simulink model "GPCA_Extension"  (Simulink 7.9)
settings: Solver=ode45  StartTime=0.0  StopTime=inf  RelTol=1e-3
PreLoadFcn:
  | GPCA_Bus_Def
InitFcn:
  | script
values from neighbouring files (symbols this model uses):
  GOutputEvents = [0 0 0 0 0 0 0 0 0 0 0 0 0 0 0 0 0 0 0 0 0]    [script.m]
  GProgrammedDoseRate = 0    [script.m]
  GProgrammedVTBI = 0    [script.m]
libraries: simulink x6
(part 2 of 3)

== stateflow chart GPCA Software Controller/StateChanger ==
  state x = displayBolusInfo [function]
    (junction 152) -> (junction 154) [order 1] : [infuStatus.isBolusInProgress == 1]{bolusing := 1; ml.GAlrmMsg = MSG_BOLUSGRANT; }
    (default) -> (junction 152)
    (junction 152) -> (junction 153) [order 2] : [infuStatus.isBolusInProgress == 0]{ml.GAlrmMsg = MSG_BOLUSDENIED; }
  state x1 = enterinto(stateId) [function]
    (junction 88) -> (junction 89) : {x1 := stateId;}
    (default) -> (junction 88) : {O_CurrentState := stateId;}
  state x = resumeInfusion [function]
    (junction 200) -> (junction 109) : {O_InfusionInProgress := 1;
        |  O_InfusionPaused := 0;
        |  O_BolusRequested := 0;}
    (default) -> (junction 199)
    (junction 199) -> (junction 200) : {infusing := 1; bolusing := 0;}
  state x = warning [function]
    (junction 127) -> (junction 108) [order 2] : [ErrCond == 17]{ml.GAlrmMsg = MSG_LOWRESR;}
    (junction 127) -> (junction 128) [order 1] : [ErrCond == 16]{ml.GAlrmMsg = MSG_FLOWRATEVARY;}
    (junction 127) -> (junction 115) [order 4] : [ErrCond == 19]{ml.GAlrmMsg = MSG_LOGERR; }
    (junction 127) -> (junction 120) [order 11] : [ErrCond == 26]{ml.GAlrmMsg = MSG_DANGERAP;}
    (junction 127) -> (junction 121) [order 3] : [ErrCond ==18]{ml.GAlrmMsg = MSG_PAUSELONG;}
    (junction 127) -> (junction 122) [order 5] : [ErrCond==20]{ml.GAlrmMsg = MSG_LOWBATT; }
    (junction 127) -> (junction 123) [order 6] : [ErrCond==21]{ml.GAlrmMsg = MSG_WRNBATTERYCHARGE;}
    (junction 127) -> (junction 125) [order 7] : [ErrCond==22]{ml.GAlrmMsg = MSG_VOLTOUTRANGE;}
    (junction 127) -> (junction 126) [order 8] : [ErrCond==23]{ml.GAlrmMsg = MSG_PUMPOVERHEAT;}
    (default) -> (junction 127) : {O_AlarmCond := ErrCond;}
    (junction 127) -> (junction 131) [order 9] : [ErrCond==24]{ml.GAlrmMsg = MSG_DANGERENVTEMP;}
    (junction 127) -> (junction 137) [order 10] : [ErrCond == 25]{ml.GAlrmMsg = MSG_DANGERHUMD;}
  state x = initInfusion [function]
    (default) -> (junction 138)
    (junction 138) -> (junction 139) : { bolusing := 0; infusing := 0; doseRate := 0; vtbi := 0;
        |   resetInfusionInstructions();}
  state x = checkDoseRate(iRate) [function]
    (junction 188) -> (junction 173) [order 2] : [iRate <= drugLibInfo.doseRateUpperHardLimit && iRate >= drugLibInfo.doseRateLowerHardLimit]
    (junction 173) -> (junction 148) [order 1] : [iRate > drugLibInfo.doseRateUpperSoftLimit || iRate < drugLibInfo.doseRateLowerSoftLimit]{ x := 1;}
    (junction 188) -> (junction 157) [order 1] : [iRate > drugLibInfo.doseRateUpperHardLimit || iRate < drugLibInfo.doseRateLowerHardLimit]{ x := 2;}
    (junction 173) -> (junction 91) [order 2] : [iRate <= drugLibInfo.doseRateUpperSoftLimit && iRate >= drugLibInfo.doseRateLowerSoftLimit]{ x:= 0;}
    (default) -> (junction 188)
  state x = clearAlrm (alrm) [function]
    (default) -> (junction 93) : {ClearCond := alrm;}
    (junction 93) -> (junction 94) : {E_AlarmClear;}
  state x = setPatientInfo [function]
    (default) -> (junction 167)
    (junction 167) -> (junction 169) : {O_PatientInfo.patientID := patientInfo.patientID;
        |  O_PatientInfo.patientAge := patientInfo.patientAge;
        |  O_PatientInfo.patientGender := patientInfo.patientGender;
        | O_PatientInfo.patientWeight := patientInfo.patientWeight;}
  state x = initPatientInfo [function]
    (junction 187) -> (junction 144) : { O_PatientInfo.patientID := 0;  O_PatientInfo.patientAge := 0;
        |   O_PatientInfo.patientGender := 0; O_PatientInfo.patientWeight := 0;}
    (default) -> (junction 187)
  state x = setDrugLibInfo [function]
    (junction 124) -> (junction 155) : { O_DrugLibInfo.drugConcentrationTypical = drugLibInfo.drugConcentrationTypical;
        |   O_DrugLibInfo.drugConcentrationUpperHardLimit = drugLibInfo.drugConcentrationUpperHardLimit;
        |   O_DrugLibInfo.drugConcentrationUpperSoftLimit = drugLibInfo.drugConcentrationUpperSoftLimit;
        |   O_DrugLibInfo.drugConcentrationLowerSoftLimit = drugLibInfo.drugConcentrationLowerSoftLimit;
        |   O_DrugLibInfo.drugConcentrationLowerHardLimit = drugLibInfo.drugConcentrationLowerHardLimit;}
    (default) -> (junction 132)
    (junction 132) -> (junction 143) : {O_DrugLibInfo.drugID = drugLibInfo.drugID; O_DrugLibInfo.amount = drugLibInfo.amount;}
    (junction 143) -> (junction 112) : { O_DrugLibInfo.doseRateTypical = drugLibInfo.doseRateTypical; O_DrugLibInfo.doseRateUnit = drugLibInfo.doseRateUnit;
        |   O_DrugLibInfo.doseRateUpperHardLimit = drugLibInfo.doseRateUpperHardLimit;
        |   O_DrugLibInfo.doseRateUpperSoftLimit = drugLibInfo.doseRateUpperSoftLimit;
        |   O_DrugLibInfo.doseRateLowerSoftLimit = drugLibInfo.doseRateLowerSoftLimit;
        |   O_DrugLibInfo.doseRateLowerHardLimit = drugLibInfo.doseRateLowerHardLimit;}
    (junction 112) -> (junction 124) : { O_DrugLibInfo.vtbiTypical = drugLibInfo.vtbiTypical; O_DrugLibInfo.vtbiUnit = drugLibInfo.vtbiUnit;
        |   O_DrugLibInfo.vtbiUpperHardLimit = drugLibInfo.vtbiUpperHardLimit;
        |   O_DrugLibInfo.vtbiUpperSoftLimit = drugLibInfo.vtbiUpperSoftLimit;
        |   O_DrugLibInfo.vtbiLowerSoftLimit = drugLibInfo.vtbiLowerSoftLimit;
        |   O_DrugLibInfo.vtbiLowerHardLimit = drugLibInfo.vtbiLowerHardLimit;}
  state x = setLOneMsg(fcond) [function]
    (default) -> (junction 98) : {O_AlarmCond := fcond;}
    (junction 98) -> (junction 99) [order 1] : [fcond==1]{ml.GAlrmMsg =MSG_OUTOFPOWER;}
    (junction 98) -> (junction 101) [order 3] : [fcond==3]{ml.GAlrmMsg = MSG_CPUFAILURE;}
    (junction 98) -> (junction 102) [order 4] : [fcond==4]{ml.GAlrmMsg = MSG_MEMORYCORRUPT;}
    (junction 98) -> (junction 103) [order 5] : [fcond==5]{ml.GAlrmMsg = MSG_PUMPTOOHOT;}
    (junction 98) -> (junction 104) [order 6] : [fcond==6]{ml.GAlrmMsg = MSG_WATCHDOGALERT;}
    (junction 98) -> (junction 100) [order 2] : [fcond==2]{ml.GAlrmMsg = MSG_REALTIMECLOCK;}
  state x = alrmLevel [function]
    (junction 96) -> (junction 184) [order 4] : [ErrCond == 0]{O_AlarmCond := ErrCond; x := 0;}
    (default) -> (junction 96)
    (junction 96) -> (junction 129) [order 1] : [ErrCond  > 0 && ErrCond <7] {O_AlarmCond := ErrCond; x:=1;}
    (junction 96) -> (junction 90) [order 2] : [ErrCond>=7 && ErrCond < 16]{O_AlarmCond := ErrCond; x:=2;}
    (junction 96) -> (junction 97) [order 3] : [ErrCond>=16]{O_AlarmCond := ErrCond; x:=3;}
  state x = setLTwoMsg(fCond) [function]
    (junction 111) -> (junction 107) [order 8] : [fCond==14]{ml.GAlrmMsg = MSG_PAUSETOOLONG;}
    (junction 111) -> (junction 105) [order 3] : [fCond==9]{ml.GAlrmMsg = MSG_OCCULUSION;}
    (junction 111) -> (junction 110) [order 9] : [fCond==15]{ml.GAlrmMsg = MSG_AIRINLINE;}
    (default) -> (junction 111) : {O_AlarmCond := fCond;}
    (junction 111) -> (junction 113) [order 1] : [fCond==7]{ml.GAlrmMsg = MSG_DOOROPEN;}
    (junction 111) -> (junction 114) [order 2] : [fCond==8]{ml.GAlrmMsg = MSG_EMPTYRESERVOIR;}
    (junction 111) -> (junction 116) [order 4] : [fCond==10]{ml.GAlrmMsg = MSG_OVERINFUSION;}
    (junction 111) -> (junction 117) [order 5] : [fCond==11]{ml.GAlrmMsg = MSG_UNDERINFUSION;}
    (junction 111) -> (junction 118) [order 6] : [fCond==12]{ml.GAlrmMsg = MSG_LESSTHANKVO;}
    (junction 111) -> (junction 119) [order 7] : [fCond==13]{ml.GAlrmMsg = MSG_RATEEXCEEDCAPACITY;}
  state x = bolusStatus [function]
    (default) -> (junction 134)
    (junction 134) -> (junction 135) [order 1] : [infuStatus.isBolusInProgress == 1]{bolusing := 1;
        | ml.GAlrmMsg = MSG_BOLUSGRANT;}
    (junction 134) -> (junction 136) [order 2] : [infuStatus.isBolusInProgress == 0]{bolusing := 0;
        | ml.GAlrmMsg = MSG_BOLUSDENIED;}
  state x = checkVTBI(inputVal) [function]
    (default) -> (junction 156)
    (junction 145) -> (junction 92) [order 2] : [(inputVal <= drugLibInfo.vtbiUpperSoftLimit) && (inputVal <= drugLibInfo.vtbiLowerSoftLimit)]{ x := 0;}
    (junction 145) -> (junction 95) [order 1] : [(inputVal > drugLibInfo.vtbiUpperSoftLimit) || (inputVal < drugLibInfo.vtbiLowerSoftLimit)]{ x := 1;}
    (junction 156) -> (junction 146) [order 1] : [(inputVal > drugLibInfo.vtbiUpperHardLimit) || (inputVal < drugLibInfo.vtbiLowerHardLimit)]{ x := 2;}
    (junction 156) -> (junction 145) [order 2] : [(inputVal <= drugLibInfo.vtbiUpperHardLimit) && (inputVal >= drugLibInfo.vtbiLowerHardLimit)]
  state x = calcFlowRate(iRate) [function]
    (junction 163) -> (junction 164) : {x := iRate /  drugInfo.drugConcentration;}
    (default) -> (junction 163)
  state x = checkDrugConcentration [function]
    (junction 174) -> (junction 172) [order 1] : [actualCon > upperHard || actualCon < lowerHard]{x := 2;}
    (junction 174) -> (junction 178) [order 2] : [actualCon <= upperHard && actualCon >= lowerHard]
    (default) -> (junction 174) : {actualCon := drugInfo.drugConcentration;
        | upperHard := drugLibInfo.drugConcentrationUpperHardLimit; upperSoft := drugLibInfo.drugConcentrationUpperSoftLimit;
        | lowerHard := drugLibInfo.drugConcentrationLowerHardLimit;  lowerSoft := drugLibInfo.drugConcentrationLowerSoftLimit;}
    (junction 178) -> (junction 176) [order 2] : [actualCon <= upperSoft && actualCon >= lowerSoft]{x := 0;}
    (junction 178) -> (junction 177) [order 1] : [actualCon > upperSoft || actualCon < lowerSoft]{x := 1;}
  state x = initDrugLib [function]
    (junction 168) -> (junction 166) : { O_DrugLibInfo.drugID := 0; O_DrugLibInfo.amount = 0; O_DrugLibInfo.diluentVolume := 0; O_DrugLibInfo.doseRateTypical := 0;
        |   O_DrugLibInfo.doseRateUpperHardLimit := 0; O_DrugLibInfo.doseRateUpperSoftLimit := 0; O_DrugLibInfo.doseRateLowerHardLimit := 0;
        |   O_DrugLibInfo.doseRateLowerSoftLimit := 0; O_DrugLibInfo.doseRateUnit := 0; O_DrugLibInfo.vtbiTypical := 0; O_DrugLibInfo.vtbiUpperHardLimit := 0;
        |   O_DrugLibInfo.vtbiUpperSoftLimit := 0; O_DrugLibInfo.vtbiLowerHardLimit := 0; O_DrugLibInfo.vtbiLowerSoftLimit := 0; O_DrugLibInfo.vtbiUnit :=0;
        |   O_DrugLibInfo.drugConcentrationTypical := 0; O_DrugLibInfo.drugConcentrationUpperHardLimit := 0; O_DrugLibInfo.drugConcentrationUpperSoftLimit := 0;
        |   O_DrugLibInfo.drugConcentrationLowerHardLimit := 0; O_DrugLibInfo.drugConcentrationLowerSoftLimit := 0;}
    (default) -> (junction 168)
  state x = init [function]
    (junction 159) -> (junction 130) : {temp := 0; tempx := 0; infusing :=0; bolusing :=0;}
    (default) -> (junction 183)
    (junction 183) -> (junction 159) : { ClearCond := 0; O_InfusionInProgress := 0; O_InfusionPaused := 0;
        |   O_BolusRequested := 0; O_ProgrammedVTBI := 0; O_ProgrammedFlowRate := 0; O_CurrentState := 0;
        |   O_AlarmCond := 0;  initDrugLib(); initPatientInfo();}
  state InfusionStateMachine
    state ConfirmPowerDown
      en: enterinto(2);
      ml.GMsgConStr := MSG_POWEROFF;
    state PowerOff
      en: enterinto(1);
      ex: ml.GMsgConStr = MSG_WELCOME;
    state POST
      en: enterinto(3);
      tempx := pumpConfigData.isPOSTSuccessful ;
    state ALM_POSTFailed
      en:  ml.GMsgConStr =MSG_POSTFAIL;
      enterinto(4);
    state InfusionInSession
      (history)
      state InfusionPaused
        en: enterinto(36);
        pauseInfusion();
        ml.GMsgConStr = MSG_INFUSIONPAUSED;
      state PausedStopConfirm
        en: ml.GMsgConStr = MSG_SPCHOOSE;
        enterinto(38);
      state InfusionStopped
        en: copyInfuStatus();
        stopInfusion();
        ml.GMsgConStr = MSG_INFUSIONSTOP;
        enterinto(39);
      state EmptyReservoir
        en: enterinto(40);
        ml.GAlrmMsg = MSG_EMPTYRESERVOIR;
      state CheckDrugWhileInfusing
        en: ml.GMsgConStr = MSG_CHECKTYPE
        enterinto(41);
        tempx := checkDrug();
      state ALMWrongDrug
        en: ml.GMsgConStr = MSG_WRONGDRUG;
        enterinto(42);
      state LevelTwoAlarming
        en: enterinto(44);
        setLTwoMsg(ErrCond);
      state InfusionSubMachine
        state Infusing
          en:  ml.GMsgConStr = MSG_INFUSING;
          enterinto(28);
          copyInfuStatus();
          on every(3, E_Clock):
          copyInfuStatus();
        state ChangeRate
          en: ml.GMsgConStr = MSG_CHANGEDR;
          ml.GSetConVal =temp;
          enterinto(30);
          copyInfuStatus();
          on every(3, E_Clock):
          copyInfuStatus();
        state CheckNewRate
          en: ml.GMsgConStr = MSG_CHECKDR;
          tempx = checkDoseRate(infuParameters.programmedDoseRate);
          temp = infuParameters.programmedDoseRate;
          enterinto(31);
          copyInfuStatus();
          on every(3, E_Clock):
          copyInfuStatus();
        state ALM_NewRateOutBound
          en: ml.GMsgConStr = MSG_ALRMDR ;
          enterinto(32);
          copyInfuStatus();
          on every(3, E_Clock):
          copyInfuStatus();
        state ConfirmStop
          en: ml.GMsgConStr = MSG_CONFIRMSTOP;
          enterinto(35);
          copyInfuStatus();
          on every(3, E_Clock):
          copyInfuStatus();
        state ConfirmPause
          en: ml.GMsgConStr = MSG_CONFIRMPAUSE;
          enterinto(34);
          copyInfuStatus();
          on every(3, E_Clock):
          copyInfuStatus();
        state BolusRequest
          en: enterinto(29);
        Infusing -> ConfirmPause [order 4] : E_PauseInfusion
        Infusing -> ChangeRate [order 2] : E_ChangeDoseRate
        ChangeRate -> Infusing [order 3] : E_Cancel
        ChangeRate -> CheckNewRate [order 2] : E_ConfirmDoseRate
        CheckNewRate -> ALM_NewRateOutBound [order 1] : [tempx>0]
        CheckNewRate -> Infusing [order 2] : [tempx==0]{setDoseRate(temp); O_ProgrammedFlowRate := calcFlowRate(temp);}
        ALM_NewRateOutBound -> Infusing [order 3] : E_Cancel
        (default) -> Infusing
        ConfirmPause -> Infusing [order 3] : E_Cancel
        ConfirmStop -> Infusing [order 3] : E_Cancel
        (junction 149) -> Infusing [order 2] : [infuStatus.isBolusInProgress == 1]{ml.GAlrmMsg = MSG_BOLUSDENIED;}
        Infusing -> (junction 149) [order 5] : E_RequestBolus
        Infusing -> ConfirmStop [order 3] : E_StopInfusion
        ALM_NewRateOutBound -> ChangeRate [order 2] : E_ChangeDoseRate
        ChangeRate -> ChangeRate [order 1] : E_Warning{warning();}
        ALM_NewRateOutBound -> ALM_NewRateOutBound [order 1] : E_Warning{warning();}
        ConfirmStop -> ConfirmStop [order 2] : E_Warning{warning();}
        Infusing -> Infusing [order 6] : E_Warning{warning();}
        ConfirmPause -> ConfirmPause [order 2] : E_Warning{warning();}
        BolusRequest -> (junction 133) : {O_BolusRequested := 0;}
        (junction 133) -> Infusing : {displayBolusInfo();}
        (junction 149) -> BolusRequest [order 1] : [infuStatus.isBolusInProgress == 0]{O_BolusRequested := 1;}
        Infusing -> Infusing [order 7] : [infusing > 0 && bolusing > 0 && infuStatus.isBolusInProgress == 0]{bolusing :=0; ml.GAlrmMsg = MSG_STOPBOLUS;}
        ChangeRate -> Infusing [order 5] : [infusionDone(vtbi) == 1]
        ALM_NewRateOutBound -> Infusing [order 5] : [infusionDone(vtbi) == 1]
        ConfirmStop -> Infusing [order 5] : [infusionDone(vtbi) == 1]
        ConfirmPause -> Infusing [order 5] : [infusionDone(vtbi) == 1]
        ConfirmPause -> ConfirmPause [order 4] : [infusing > 0 && bolusing > 0 && infuStatus.isBolusInProgress == 0]{bolusing :=0; ml.GAlrmMsg = MSG_STOPBOLUS;}
        ConfirmStop -> ConfirmStop [order 4] : [infusing > 0 && bolusing > 0 && infuStatus.isBolusInProgress == 0]
            | {bolusing :=0; ml.GAlrmMsg = MSG_STOPBOLUS;}
        ChangeRate -> ChangeRate [order 4] : [infusing > 0 && bolusing > 0 && infuStatus.isBolusInProgress == 0]
            | {bolusing :=0; ml.GAlrmMsg = MSG_STOPBOLUS;}
        ALM_NewRateOutBound -> ALM_NewRateOutBound [order 4] : [infusing > 0 && bolusing > 0 && infuStatus.isBolusInProgress == 0]
            | {bolusing :=0; ml.GAlrmMsg = MSG_STOPBOLUS;}
      state PausedTooLong
        en: enterinto(37);
        ml.GAlrmMsg = MSG_PAUSETOOLONG;
      InfusionPaused -> LevelTwoAlarming [order 5] : [alrmLevel()==2]{pauseInfusion();}
      InfusionPaused -> PausedTooLong [order 1] : E_Alarm[ErrCond == 13]
      InfusionPaused -> PausedStopConfirm [order 3] : E_StopInfusion
      PausedStopConfirm -> InfusionPaused [order 3] : E_Cancel
      PausedStopConfirm -> InfusionStopped [order 1] : E_ConfirmStopInfusion
      EmptyReservoir -> CheckDrugWhileInfusing [order 2] : E_CheckDrug
      CheckDrugWhileInfusing -> ALMWrongDrug [order 1] : [tempx > 0]
      EmptyReservoir -> InfusionStopped [order 3] : E_StopInfusion
      ALMWrongDrug -> InfusionStopped [order 1] : E_StopInfusion
      LevelTwoAlarming -> EmptyReservoir [order 4] : [ErrCond==7]
      (default) -> InfusionSubMachine
      InfusionSubMachine -> LevelTwoAlarming : [alrmLevel()==2]{pauseInfusion();}
      LevelTwoAlarming -> InfusionStopped [order 2] : E_StopInfusion{clearLevel2Alarm();}
      ALMWrongDrug -> ALMWrongDrug [order 3] : E_Warning{warning();}
      PausedStopConfirm -> LevelTwoAlarming [order 4] : [alrmLevel()==2]{pauseInfusion();}
      ALMWrongDrug -> CheckDrugWhileInfusing [order 2] : E_CheckDrug
      LevelTwoAlarming -> LevelTwoAlarming [order 1] : E_Warning{warning();}
      EmptyReservoir -> EmptyReservoir [order 1] : E_Warning{warning();}
      InfusionStopped -> InfusionStopped [order 2] : E_Warning{warning();}
      InfusionPaused -> InfusionPaused [order 2] : E_Warning{warning();}
      PausedStopConfirm -> PausedStopConfirm [order 2] : E_Warning{warning();}
      PausedTooLong -> PausedTooLong [order 2] : E_Warning{warning();}
      PausedTooLong -> InfusionStopped [order 1] : E_StopInfusion
      Infusing -> InfusionStopped [order 1] : [infusionDone(vtbi) == 1]
          | {ml.GAlrmMsg = MSG_BLANK;}
      InfusionPaused -> Infusing [order 4] : E_Cancel{resumeInfusion();}
      CheckDrugWhileInfusing -> Infusing [order 2] : [tempx == 0]{resumeInfusion();}
      LevelTwoAlarming -> Infusing [order 3] : E_ClearAlarm{clearLevel2Alarm(); resumeInfusion();}
      PausedTooLong -> Infusing [order 3] : E_ClearAlarm{ClearCond:=13; resumeInfusion();E_AlarmClear}
      ConfirmStop -> InfusionStopped [order 1] : E_ConfirmStopInfusion{ml.GAlrmMsg = MSG_BLANK;}
      ConfirmPause -> InfusionPaused [order 1] : E_ConfirmPauseInfusion{ml.GAlrmMsg = MSG_BLANK;}
    state Init
    state POSTDONE
      en: ml.GMsgConStr = MSG_POSTDONE;
      enterinto(45);
      tempx = 0;
    state LEVELONEALRM
      en: setLOneMsg(ErrCond);
      enterinto(43);
    state CheckDrugRoutine
      (history)
      state CheckAdminSet
        en: enterinto(5);
        ml.GMsgConStr =MSG_ADMINCHECK;
        tempx := pumpConfigData.isAdminSetCheckPassed;
      state CheckPrime
        en:  enterinto(7);
        tempx = 0;
        ml.GMsgConStr = MSG_PRIME;
        tempx = pumpConfigData.isPumpPrimed;
      state ALM_WrongAdminCheck
        en: enterinto(6);
        ml.GMsgConStr = MSG_ADMINFAIL;
      state PrimeFailed
        en: enterinto(8);
        ml.GMsgConStr = MSG_PRIMEFAIL;
      state DisplayDrugInfo
        en: enterinto(9);
        tempx = 0;
        ml.GMsgConStr = MSG_DRUGINFO;
      state CheckDrug_CheckType
        en: enterinto(10);
        ml.GMsgConStr = MSG_CHECKTYPE;
        tempx := checkDrugType();
      state UnknownDrug
        en: enterinto(11);
        ml.GMsgConStr =MSG_WRONGDRUG;
      state Check_DrugUnits
        en: enterinto(12);
        ml.GMsgConStr = MSG_CHECKDU;
        tempx := checkDrugUnits();
      state IncorrectDrugUnits
        en: enterinto(13);
        ml.GMsgConStr =MSG_WRONGDU;
      state Check_Concen
        en:enterinto(14);
        ml.GMsgConStr = MSG_CHECKCON;
        tempx := checkDrugConcentration();
      state WrongConcentration
        en: enterinto(15);
        ml.GMsgConStr = MSG_WRONGCON;
      state WRN_DangerCon
        en: enterinto(16);
        ml.GMsgConStr = MSG_DANGECON;
      state DisplayPatientProfile
        en:   enterinto(18);
        ml.GMsgConStr = MSG_PATIENTINFO;
      UnknownDrug -> CheckDrug_CheckType [order 2] : E_CheckDrug
      Check_Concen -> WrongConcentration [order 1] : [tempx==2]
      Check_DrugUnits -> IncorrectDrugUnits [order 1] : [tempx!=0]
      IncorrectDrugUnits -> CheckDrug_CheckType [order 1] : E_CheckDrug
      Check_DrugUnits -> Check_Concen [order 2] : [tempx==0]
      CheckDrug_CheckType -> UnknownDrug [order 1] : [tempx==1]
      CheckDrug_CheckType -> Check_DrugUnits [order 2] : [tempx==0]
      Check_Concen -> WRN_DangerCon [order 2] : [tempx==1]
      Check_Concen -> DisplayPatientProfile [order 3] : [tempx==0]{setPatientInfo();}
      WRN_DangerCon -> DisplayPatientProfile [order 2] : E_ConfirmConcentration{setPatientInfo();}
      ALM_WrongAdminCheck -> CheckAdminSet [order 2] : E_CheckAdminSet
      CheckAdminSet -> ALM_WrongAdminCheck [order 1] : [tempx==0]
      CheckAdminSet -> CheckPrime [order 2] : [tempx==1]{E_Restart; }
      PrimeFailed -> CheckPrime [order 2] : E_Prime
      CheckPrime -> PrimeFailed [order 1] : [tempx==0]
      CheckPrime -> DisplayDrugInfo [order 2] : [tempx==1]{setDrugLibInfo();}
      DisplayPatientProfile -> DisplayDrugInfo [order 3] : E_Cancel
      DisplayDrugInfo -> CheckDrug_CheckType [order 1] : E_CheckDrug
      ALM_WrongAdminCheck -> ALM_WrongAdminCheck [order 1] : E_Warning{warning();}
      UnknownDrug -> UnknownDrug [order 1] : E_Warning{warning();}
      WrongConcentration -> CheckDrug_CheckType [order 1] : E_CheckDrug
      WrongConcentration -> WrongConcentration [order 2] : E_Warning{warning();}
      DisplayDrugInfo -> DisplayDrugInfo [order 2] : E_Warning{warning();}
      WRN_DangerCon -> WRN_DangerCon [order 3] : E_Warning{warning();}
      WRN_DangerCon -> CheckDrug_CheckType [order 1] : E_CheckDrug
      DisplayPatientProfile -> DisplayPatientProfile [order 2] : E_Warning{warning();}
      PrimeFailed -> PrimeFailed [order 1] : E_Warning{warning();}
      IncorrectDrugUnits -> IncorrectDrugUnits [order 2] : E_Warning{warning();}
    state ConfigureInfusionProgram
      (history)
      state ALM_VTBIOutBound
        en: enterinto(22);
        ml.GMsgConStr = MSG_ALMVTBI;
      state DisplayDoseRate
        en:  enterinto(23);
        ml.GMsgConStr = MSG_DISPLAYDR;
        tempx = 0;
        setDoseRate(drugLibInfo.doseRateTypical);
      state DisplayVTBI
        en:   enterinto(19);
        ml.GMsgConStr = MSG_VTBI;
        setVTBI(drugLibInfo.vtbiTypical);
      state ChangeVTBI
        en: enterinto(20);
        ml.GMsgConStr = MSG_CHANGEVTBI;
      state CheckVTBI
        en: enterinto(21);
        ml.GMsgConStr = MSG_CHECKVTBI;
        tempx := checkVTBI(infuParameters.programmedVTBI);
      state ChangeDoseRate
        en: enterinto(24);
        ml.GMsgConStr = MSG_CHANGEDR;
      state CheckDoseRate
        en: enterinto(25);
        ml.GMsgConStr = MSG_CHECKDR;
        tempx := checkDoseRate(infuParameters.programmedDoseRate);
      state ALM_DoseRateOutBound
        en: enterinto(26);
        ml.GMsgConStr = MSG_ALRMDR;
      state DisplaySettings
        en: enterinto(27);
        ml.GMsgConStr = MSG_DISPLAYSET;
      state ReadyToStart
        en: enterinto(48);
      state WRN_VTBIOutBound
        en: enterinto(46);
        ml.GMsgConStr = MSG_WRNVTBI;
      state WRN_DOSERATEOUTSOFTLIMITS
        en:  enterinto(47);
        ml.GMsgConStr = MSG_WRNDR;
      CheckVTBI -> ALM_VTBIOutBound [order 3] : [tempx==2]
      ALM_VTBIOutBound -> ChangeVTBI [order 2] : E_ChangeVTBI
      CheckVTBI -> DisplayDoseRate [order 2] : [tempx==0]{setVTBI(infuParameters.programmedVTBI);}
      ChangeVTBI -> CheckVTBI [order 1] : E_ConfirmVTBI
      DisplayVTBI -> ChangeVTBI [order 1] : E_ChangeVTBI
      ChangeVTBI -> DisplayVTBI [order 2] : E_Cancel
      DisplayVTBI -> DisplayDoseRate [order 2] : E_ConfirmVTBI
      DisplayDoseRate -> ChangeDoseRate [order 1] : E_ChangeDoseRate
      ChangeDoseRate -> DisplayDoseRate [order 3] : E_Cancel
      ChangeDoseRate -> CheckDoseRate [order 1] : E_ConfirmDoseRate
      CheckDoseRate -> ALM_DoseRateOutBound [order 3] : [tempx==2]
      ALM_DoseRateOutBound -> ChangeDoseRate [order 2] : E_ChangeDoseRate
      CheckDoseRate -> DisplaySettings [order 2] : [tempx==0]{setDoseRate(infuParameters.programmedDoseRate);}
      DisplayDoseRate -> DisplaySettings [order 2] : E_ConfirmDoseRate
      DisplaySettings -> ReadyToStart [order 1] : E_StartInfusion{E_RequestToStart}
      DisplaySettings -> DisplaySettings [order 3] : E_Warning{warning();}
      WRN_VTBIOutBound -> WRN_VTBIOutBound [order 1] : E_Warning{warning();}
      ReadyToStart -> ReadyToStart [order 2] : E_Warning{warning();}
      DisplayVTBI -> DisplayVTBI [order 3] : E_Warning{warning();}
      ReadyToStart -> DisplaySettings [order 3] : E_NotReady{ml.GAlrmMsg = MSG_NOTREADY;}
      DisplaySettings -> DisplayVTBI [order 2] : E_ConfigureInfusionProgram
      ChangeDoseRate -> ChangeDoseRate [order 2] : E_Warning{warning();}
      CheckVTBI -> WRN_VTBIOutBound [order 1] : [tempx==1]
      WRN_VTBIOutBound -> DisplayDoseRate [order 2] : E_ConfirmVTBI{setVTBI(infuParameters.programmedVTBI);}
      WRN_VTBIOutBound -> ChangeVTBI [order 3] : E_ChangeVTBI
      WRN_DOSERATEOUTSOFTLIMITS -> DisplaySettings [order 1] : E_ConfirmDoseRate{setDoseRate(infuParameters.programmedDoseRate);}
      CheckDoseRate -> WRN_DOSERATEOUTSOFTLIMITS [order 1] : [tempx==1]
      DisplayDoseRate -> DisplayDoseRate [order 3] : E_Warning{warning();}
      ALM_DoseRateOutBound -> ALM_DoseRateOutBound [order 1] : E_Warning{warning();}
      ALM_VTBIOutBound -> ALM_VTBIOutBound [order 1] : E_Warning{warning();}
      ChangeVTBI -> ChangeVTBI [order 3] : E_Warning{warning();}
      WRN_DOSERATEOUTSOFTLIMITS -> ChangeDoseRate [order 2] : E_ChangeDoseRate
    Init -> PowerOff
    ALM_POSTFailed -> PowerOff [order 1] : E_PowerButton
    PowerOff -> POST : E_PowerButton{init(); ml.GMsgConStr = MSG_POST;}
    ConfirmPowerDown -> CheckDrugRoutine [order 3] : E_Cancel[tempx==1]
    InfusionInSession -> ConfirmPowerDown [order 1] : E_PowerButton{tempx=3;}
    POSTDONE -> POSTDONE [order 3] : E_Warning{warning();}
    ConfirmPowerDown -> PowerOff [order 6] : E_ConfirmPowerDown{O_AlarmCond := 0; ml.GAlrmMsg := MSG_BLANK;}
    ConfirmPowerDown -> ConfigureInfusionProgram [order 2] : E_Cancel[tempx==2]
    ConfigureInfusionProgram -> ConfirmPowerDown [order 1] : E_PowerButton{tempx=2;}
    ConfirmPowerDown -> InfusionInSession [order 1] : E_Cancel[tempx==3]
    InfusionInSession -> LEVELONEALRM [order 2] : [alrmLevel()==1]{resetInfusionInstructions();}
    InfusionStopped -> CheckAdminSet [order 1] : E_NewInfusion{resetInfusionInstructions(); initInfuStatus();}
    POSTDONE -> CheckAdminSet [order 2] : E_CheckAdminSet{resetInfusionInstructions(); initInfuStatus();}
    ConfirmPowerDown -> ConfirmPowerDown [order 5] : E_Warning{warning();}
    ALM_POSTFailed -> ALM_POSTFailed [order 2] : E_Warning{warning();}
    POST -> ALM_POSTFailed [order 2] : [tempx==0]
    CheckDrugRoutine -> LEVELONEALRM [order 2] : [alrmLevel()==1]
    (default) -> Init
    ConfigureInfusionProgram -> LEVELONEALRM [order 2] : [alrmLevel()==1]
    LEVELONEALRM -> PowerOff : E_PowerButton
        | {O_AlarmCond := 0;
        | ml.GAlrmMsg := MSG_BLANK;}
    POSTDONE -> ConfirmPowerDown [order 1] : E_PowerButton{tempx=4;}
    ConfirmPowerDown -> POSTDONE [order 4] : E_Cancel[tempx==4]
    POST -> POSTDONE [order 1] : [tempx==1]
    DisplayPatientProfile -> DisplayVTBI [order 1] : E_ConfigureInfusionProgram{setDrugLibInfo();}
    ReadyToStart -> Infusing [order 1] : E_Ready {startInfusion();}
    CheckDrugRoutine -> ConfirmPowerDown [order 1] : E_PowerButton{tempx=1;}
  state x = infusionDone(expectedVolume) [function]
    (default) -> (junction 106) : {x:=0;}
    (junction 106) -> (junction 141) [order 2] : [infuStatus.totalVolumeInfused < expectedVolume]{x := 0;}
    (junction 106) -> (junction 142) [order 1] : [infuStatus.totalVolumeInfused >= expectedVolume]{x := 1;}
  state x = clearLevel2Alarm [function]
    (junction 185) -> (junction 186) : {ml.GAlrmMsg = MSG_BLANK; E_AlarmClear;}
    (default) -> (junction 185)
  state x = checkDrugType [function]
    (junction 181) -> (junction 175) [order 2] : [drugInfo.drugDoseAmount == drugLibInfo.amount]{x := 0;}
    (junction 181) -> (junction 171) [order 1] : [drugInfo.drugDoseAmount != drugLibInfo.amount]{x := 1;}
    (default) -> (junction 182)
    (junction 182) -> (junction 147) [order 1] : [drugInfo.drugID != drugLibInfo.drugID]{x:=1;}
    (junction 182) -> (junction 181) [order 2] : [drugInfo.drugID == drugLibInfo.drugID]
  state x = checkDrug [function]
    (junction 162) -> (junction 161) [order 1] : [flag == 1]{x := 1;}
    (default) -> (junction 162) : {flag := checkDrugType();}
    (junction 192) -> (junction 140) [order 1] : [flag == 1]{x := 1;}
    (junction 192) -> (junction 189) [order 2] : [flag == 0]{flag:= checkDrugConcentration();}
    (junction 189) -> (junction 191) [order 2] : [flag == 0]{x := 0;}
    (junction 189) -> (junction 190) [order 1] : [flag > 0]{x := 1;}
    (junction 162) -> (junction 192) [order 2] : [flag == 0]{flag := checkDrugUnits();}
  state x = checkDrugUnits [function]
    (junction 150) -> (junction 158) [order 2] : [drugInfo.drugVolumeUnit == drugLibInfo.vtbiUnit]{ x:= 0;}
    (default) -> (junction 170)
    (junction 150) -> (junction 160) [order 1] : [drugInfo.drugVolumeUnit != drugLibInfo.vtbiUnit]{x := 1;}
    (junction 170) -> (junction 150) [order 2] : [drugInfo.drugDoseUnit == drugLibInfo.doseRateUnit]
    (junction 170) -> (junction 151) [order 1] : [drugInfo.drugDoseUnit != drugLibInfo.doseRateUnit]{x := 1;}
  state x = stopInfusion [function]
    (junction 194) -> (junction 193) : {O_ProgrammedVTBI := 0;
        |  O_ProgrammedFlowRate := 0;}
    (junction 209) -> (junction 194) : {O_InfusionInProgress := 0;
        |  O_InfusionPaused := 0;
        |  O_BolusRequested := 0;}
    (default) -> (junction 208)
    (junction 208) -> (junction 209) : {infusing := 0; bolusing := 0;}
  state x = setVTBI(iVTBI) [function]
    (default) -> (junction 195)
    (junction 195) -> (junction 196) : {vtbi := iVTBI;}
  state x = setDoseRate(iRate) [function]
    (default) -> (junction 197)
    (junction 197) -> (junction 198) : {doseRate := iRate;}
  state x = startInfusion [function]
    (default) -> (junction 201)
    (junction 201) -> (junction 202) : {O_ProgrammedFlowRate := calcFlowRate(doseRate);
        |  O_ProgrammedVTBI := vtbi;}
    (junction 202) -> (junction 203) : {O_InfusionInProgress := 1;
        |  O_InfusionPaused := 0;
        |  O_BolusRequested := 0;}
    (junction 203) -> (junction 204) : {infusing := 1; bolusing := 0;}
  state x = pauseInfusion [function]
    (default) -> (junction 205)
    (junction 205) -> (junction 206) : {infusing := 0; bolusing := 0;}
    (junction 206) -> (junction 207) : {O_InfusionInProgress := 1;
        |  O_InfusionPaused := 1;
        |  O_BolusRequested := 0;}
  state x = resetInfusionInstructions [function]
    (junction 211) -> (junction 210) : {stopInfusion();}
    (default) -> (junction 211)
  state x = copyInfuStatus [function]
    (default) -> (junction 212)
    (junction 212) -> (junction 213) : {O_InfuStatus.isBolusInProgress := infuStatus.isBolusInProgress;
        |  O_InfuStatus.totalVolumeInfused := infuStatus.totalVolumeInfused;
        |  O_InfuStatus.remainingVolumeInReservoir := infuStatus.remainingVolumeInReservoir;}
  state x = initInfuStatus [function]
    (default) -> (junction 214)
    (junction 214) -> (junction 215) : {O_InfuStatus.isBolusInProgress := 0;
        |  O_InfuStatus.totalVolumeInfused := 0;
        |  O_InfuStatus.remainingVolumeInReservoir := infuStatus.remainingVolumeInReservoir;}
  state x = outputInfuStatus(a,b,c) [function]
    (default) -> (junction 216)
    (junction 216) -> (junction 217) : {O_InfuStatus.isBolusInProgress := a;
        |  O_InfuStatus.totalVolumeInfused := b;
        |  O_InfuStatus.remainingVolumeInReservoir := c;}
  data: x function_output double; stateId function_input uint32; x1 function_output uint32; x function_output double; x function_output uint32; x function_output uint32; iRate function_input double; x function_output uint32; alrm function_input uint32; x function_output uint32; x function_output double; x function_output double; x function_output double; fcond function_input uint32; x function_output uint32; x function_output uint32; fCond function_input uint32; x function_output uint32; x function_output uint32; inputVal function_input double; x function_output uint32; x function_output double; iRate function_input double; x function_output double; actualCon temporary double; upperHard temporary double; upperSoft temporary double; lowerHard temporary double; lowerSoft temporary double; x function_output double; x function_output double; expectedVolume function_input double; x function_output double; x function_output uint32; x function_output uint32; x function_output double; flag temporary boolean; x function_output double; x function_output double; iVTBI function_input double; x function_output double; iRate function_input double; x function_output double; x function_output double; x function_output double; x function_output double; x function_output double; x function_output double; x function_output double; a function_input double; b function_input double; c function_input double; ErrCond input double; ClearCond output uint32; O_InfusionInProgress output boolean; O_InfusionPaused output boolean; O_BolusRequested output boolean; O_ProgrammedVTBI output double; O_ProgrammedFlowRate output double; MSG_WELCOME constant uint32 =1; MSG_POWEROFF constant uint32 =2; MSG_POST constant uint32 =3; MSG_POSTFAIL constant uint32 =4; MSG_ADMINCHECK constant uint32 =5; MSG_ADMINFAIL constant uint32 =6; MSG_PRIME constant uint32 =7; MSG_PRIMEFAIL constant uint32 =8; MSG_CHECKTYPE constant uint32 =9; MSG_WRONGDRUG constant uint32 =10; MSG_CHECKDU constant uint32 =11; MSG_WRONGDU constant uint32 =12; MSG_CHECKCON constant uint32 =13; MSG_WRONGCON constant uint32 =14; MSG_DANGECON constant uint32 =15; MSG_PATIENTINFO constant uint32 =16; MSG_CHANGEVTBI constant uint32 =18; MSG_VTBI constant uint32 =17; MSG_CHECKVTBI constant uint32 =19; MSG_ALMVTBI constant uint32 =20; MSG_DISPLAYDR constant uint32 =21; MSG_CHECKDR constant uint32 =22; MSG_CHANGEDR constant uint32 =23; MSG_DISPLAYSET constant uint32 =24; MSG_ALRMDR constant uint32 =25; MSG_INFUSING constant uint32 =26; MSG_DANGERENVTEMP constant uint32 =24; MSG_DANGERHUMD constant uint32 =25; MSG_DANGERAP constant uint32 =26; MSG_POSTDONE constant uint32 =27; MSG_DRUGINFO constant uint32 =28; MSG_BOLUSGRANT constant uint32 =28; MSG_BOLUSDENIED constant uint32 =29; MSG_STOPBOLUS constant uint32 =30; MSG_EMPTYRESERVOIR constant uint32 =8; MSG_DOOROPEN constant uint32 =7; MSG_AIRINLINE constant uint32 =15; MSG_OCCULUSION constant uint32 =9; MSG_PAUSETOOLONG constant uint32 =14; MSG_FLOWRATEVARY constant uint32 =16; MSG_OVERINFUSION constant uint32 =10; MSG_UNDERINFUSION constant uint32 =11; MSG_LESSTHANKVO constant uint32 =12; MSG_RATEEXCEEDCAPACITY constant uint32 =13; MSG_REALTIMECLOCK constant uint32 =2; MSG_WATCHDOGALERT constant uint32 =6; MSG_OUTOFPOWER constant uint32 =1; MSG_MEMORYCORRUPT constant uint32 =4; MSG_CPUFAILURE constant uint32 =3; MSG_INFUSIONSTOP constant uint32 =29; MSG_SPCHOOSE constant uint32 =30; MSG_INFUSIONPAUSED constant uint32 =31; MSG_CONFIRMPAUSE constant uint32 =32; MSG_CONFIRMSTOP constant uint32 =33; MSG_STOPPAUSE constant uint32 =34; MSG_LOGERR constant uint32 =19; MSG_LOWBATT constant uint32 =20; MSG_LOWRESR constant uint32 =17; MSG_WRNDR constant uint32 =35; MSG_WRNVTBI constant uint32 =36; temp local double; MSG_NOTREADY constant uint32 =27; MSG_BLANK constant uint32 =31; MSG_WRNBATTERYCHARGE constant uint32 =21; MSG_VOLTOUTRANGE constant uint32 =22; O_CurrentState output uint32; tempx local uint32; drugLibInfo input Bus: DrugLibrary size=1; patientInfo input Bus: PatientInformation size=1; drugInfo input Bus: DrugInformation size=1; infuParameters input Bus: InfusionParameters size=1; infuStatus input Bus: InfusionStatus size=1; pumpConfigData input Bus: PumpConfigurationsStatus size=1; O_DrugLibInfo output Bus: DrugLibrary size=1; O_PatientInfo output Bus: PatientInformation size=1; O_InfuStatus output Bus: InfusionStatus size=1; O_AlarmCond output uint32; infusing local boolean; bolusing local boolean; vtbi local double; doseRate local double; initDrugReservoirVolume local double; MSG_PUMPTOOHOT constant uint32 =5; MSG_PAUSELONG constant uint32 =18; MSG_PUMPOVERHEAT constant uint32 =23; MSG_DISPINFU constant uint32 =32
  events: E_Clock input EITHER_EDGE_EVENT; E_Restart output EITHER_EDGE_EVENT; E_AlarmClear output EITHER_EDGE_EVENT; E_RequestToStart output EITHER_EDGE_EVENT; E_Alarm input RISING_EDGE_EVENT; E_Warning input RISING_EDGE_EVENT; E_Ready input RISING_EDGE_EVENT; E_NotReady input RISING_EDGE_EVENT; E_StartSimulation input RISING_EDGE_EVENT; E_PowerButton input RISING_EDGE_EVENT; E_NewInfusion input RISING_EDGE_EVENT; E_CheckAdminSet input RISING_EDGE_EVENT; E_Prime input RISING_EDGE_EVENT; E_CheckDrug input RISING_EDGE_EVENT; E_ConfigureInfusionProgram input RISING_EDGE_EVENT; E_ConfirmConcentration input RISING_EDGE_EVENT; E_ConfirmDoseRate input RISING_EDGE_EVENT; E_ConfirmVTBI input RISING_EDGE_EVENT; E_StartInfusion input RISING_EDGE_EVENT; E_ChangeDoseRate input RISING_EDGE_EVENT; E_ChangeVTBI input RISING_EDGE_EVENT; E_PauseInfusion input RISING_EDGE_EVENT; E_ConfirmPauseInfusion input RISING_EDGE_EVENT; E_StopInfusion input RISING_EDGE_EVENT; E_ConfirmStopInfusion input RISING_EDGE_EVENT; E_RequestBolus input RISING_EDGE_EVENT; E_ClearAlarm input RISING_EDGE_EVENT; E_ConfirmPowerDown input RISING_EDGE_EVENT; E_Cancel input RISING_EDGE_EVENT

== stateflow chart WebSocketsBridge/Converter ==
  note: Do not put any code along
      | the transitions that run
      | down the right side!
  state st0
  (junction 702) -> (junction 694) [order 1] : [CommandID == 2]
  (junction 694) -> (junction 695) : { PowerButton = 1; }
  (junction 695) -> (junction 703)
  (junction 703) -> (junction 709)
  (junction 704) -> (junction 697) [order 1] : [CommandID == 3]
  (junction 697) -> (junction 696) : { StartNewInfusion = 1; }
  (junction 696) -> (junction 709)
  (junction 702) -> (junction 704) [order 2]
  (junction 704) -> (junction 705) [order 2]
  (junction 709) -> (junction 710)
  (junction 705) -> (junction 700) [order 1] : [CommandID == 4]
  (junction 700) -> (junction 701) : { CheckAdminSet = 1; }
  (junction 701) -> (junction 710)
  (junction 705) -> (junction 706) [order 2]
  (junction 710) -> (junction 711)
  (junction 706) -> (junction 699) [order 1] : [CommandID == 5]
  (junction 699) -> (junction 698) : { Prime = 1; }
  (junction 698) -> (junction 711)
  (default) -> st0 : /* Converts Command IDs received from the GPCA-UI
      |     into Events for the GPCA Controller */
  st0 -> (junction 779) : { StartStopSimulation = 0; PowerButton = 0; StartNewInfusion = 0; CheckAdminSet = 0; Prime = 0; CheckDrug = 0;
      |   ConfigureInfusionProgram = 0; ConfirmConcentration = 0; ConfirmDoseRate = 0; ConfirmVTBI = 0; StartInfusion = 0;
      |   ChangeDoseRate = 0; ChangeVTBI = 0; StartInfusion = 0; ChangeDoseRate = 0; ChangeVTBI = 0; PauseInfusion = 0;
      |   ConfirmPauseInfusion = 0; StopInfusion = 0; ConfirmStopInfusion = 0; RequestBolus = 0; ClearAlarm = 0;
      |   ConfirmPowerDown = 0; Cancel = 0; }
  (junction 770) -> (junction 769) [order 2]
  (junction 708) -> (junction 707)
  (junction 713) -> (junction 716)
  (junction 714) -> (junction 713) : { CheckDrug = 1; }
  (junction 715) -> (junction 714) [order 1] : [CommandID == 6]
  (junction 706) -> (junction 715) [order 2]
  (junction 711) -> (junction 716)
  (junction 718) -> (junction 717) : { ConfigureInfusionProgram = 1; }
  (junction 717) -> (junction 720)
  (junction 719) -> (junction 718) [order 1] : [CommandID == 7]
  (junction 715) -> (junction 719) [order 2]
  (junction 716) -> (junction 720)
  (junction 722) -> (junction 721) : { ConfirmConcentration = 1; }
  (junction 721) -> (junction 724)
  (junction 723) -> (junction 722) [order 1] : [CommandID == 8]
  (junction 719) -> (junction 723) [order 2]
  (junction 720) -> (junction 724)
  (junction 733) -> (junction 725) [order 1] : [CommandID == 9]
  (junction 725) -> (junction 726) : { ConfirmDoseRate = 1; }
  (junction 726) -> (junction 734)
  (junction 734) -> (junction 738)
  (junction 735) -> (junction 728) [order 1] : [CommandID == 10]
  (junction 728) -> (junction 727) : { ConfirmVTBI = 1; }
  (junction 727) -> (junction 738)
  (junction 733) -> (junction 735) [order 2]
  (junction 735) -> (junction 736) [order 2]
  (junction 738) -> (junction 739)
  (junction 736) -> (junction 731) [order 1] : [CommandID == 11]
  (junction 731) -> (junction 732) : { StartInfusion = 1; }
  (junction 732) -> (junction 739)
  (junction 736) -> (junction 737) [order 2]
  (junction 739) -> (junction 740)
  (junction 737) -> (junction 730) [order 1] : [CommandID == 12]
  (junction 730) -> (junction 729) : { ChangeDoseRate = 1; }
  (junction 729) -> (junction 740)
  (junction 748) -> (junction 752)
  (junction 743) -> (junction 742) [order 1] : [CommandID == 13]
  (junction 742) -> (junction 741) : { ChangeVTBI = 1; }
  (junction 741) -> (junction 744)
  (junction 737) -> (junction 743) [order 2]
  (junction 740) -> (junction 744)
  (junction 747) -> (junction 746) [order 1] : [CommandID == 14]
  (junction 746) -> (junction 745) : { PauseInfusion = 1; }
  (junction 745) -> (junction 748)
  (junction 743) -> (junction 747) [order 2]
  (junction 744) -> (junction 748)
  (junction 751) -> (junction 750) [order 1] : [CommandID == 15]
  (junction 750) -> (junction 749) : { ConfirmPauseInfusion = 1; }
  (junction 749) -> (junction 752)
  (junction 747) -> (junction 751) [order 2]
  (junction 723) -> (junction 733) [order 2]
  (junction 724) -> (junction 734)
  (junction 780) -> (junction 703)
  (junction 757) -> (junction 755) [order 1] : [CommandID == 16]
  (junction 755) -> (junction 756) : { StopInfusion = 1; }
  (junction 756) -> (junction 759)
  (junction 757) -> (junction 758) [order 2]
  (junction 759) -> (junction 760)
  (junction 758) -> (junction 754) [order 1] : [CommandID == 17]
  (junction 754) -> (junction 753) : { ConfirmStopInfusion = 1; }
  (junction 753) -> (junction 760)
  (junction 763) -> (junction 762) [order 1] : [CommandID == 18]
  (junction 762) -> (junction 761) : { RequestBolus = 1; }
  (junction 761) -> (junction 764)
  (junction 758) -> (junction 763) [order 2]
  (junction 760) -> (junction 764)
  (junction 767) -> (junction 766) [order 1] : [CommandID == 19]
  (junction 766) -> (junction 765) : { ClearAlarm = 1; }
  (junction 765) -> (junction 768)
  (junction 763) -> (junction 767) [order 2]
  (junction 764) -> (junction 768)
  (junction 770) -> (junction 712) [order 1] : [CommandID == 20]
  (junction 712) -> (junction 708) : { ConfirmPowerDown = 1; }
  (junction 767) -> (junction 770) [order 2]
  (junction 768) -> (junction 707)
  (junction 751) -> (junction 757) [order 2]
  (junction 769) -> (junction 771) [order 1] : [CommandID == 21]
  (junction 771) -> (junction 775) : { Cancel = 1; }
  (junction 774) -> (junction 772)
  (junction 707) -> (junction 773)
  (junction 769) -> (junction 772) [order 2]
  (junction 775) -> (junction 773)
  (junction 773) -> (junction 774)
  (junction 772) -> (junction 776)
  (junction 752) -> (junction 759)
  (junction 779) -> (junction 777) [order 1] : [CommandID == 1]
  (junction 777) -> (junction 778) : { StartStopSimulation = 1; }
  (junction 778) -> (junction 780)
  (junction 779) -> (junction 702) [order 2]
  data: CommandID input int32 size=1; StartStopSimulation output double; PowerButton output double; StartNewInfusion output double; CheckAdminSet output double; Prime output double; CheckDrug output double; ConfigureInfusionProgram output double; ConfirmConcentration output double; ConfirmDoseRate output double; ConfirmVTBI output double; StartInfusion output double; ChangeDoseRate output double; ChangeVTBI output double; PauseInfusion output double; ConfirmPauseInfusion output double; StopInfusion output double; ConfirmStopInfusion output double; RequestBolus output double; ClearAlarm output double; ConfirmPowerDown output double; Cancel output double
